simulink model "generic_IVS"  (R2024a)
settings: Solver=FixedStepDiscrete  StartTime=0.0  StopTime=inf  FixedStep=0.001  RelTol=1e-3  EnableMultiTasking=on
libraries: CarMaker4SL x57, simulink x1, slpidlib x1
(part 3 of 4)

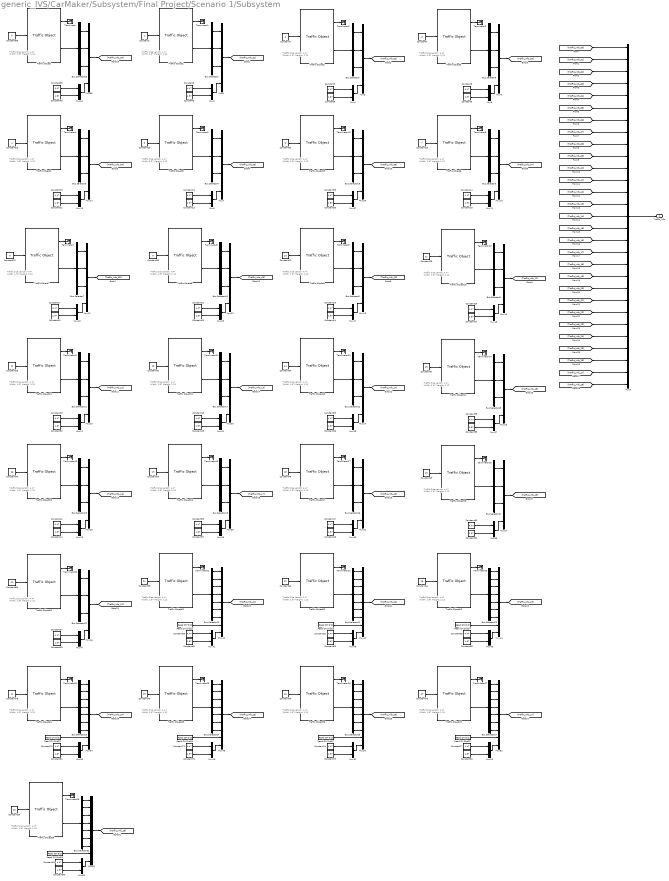
== system generic_IVS/CarMaker/Subsystem/Final Project/Scenario 1/Subsystem ==
  note: Traffic Size
      | Length: 4.47
      | Width: 1.97
      | Height: 1.12
  note: Traffic Size
      | Length: 4.47
      | Width: 1.97
      | Height: 1.12
  note: Traffic Size
      | Length: 4.47
      | Width: 1.97
      | Height: 1.12
  note: Traffic Size
      | Length: 4.47
      | Width: 1.97
      | Height: 1.12
  note: Traffic Size
      | Length: 4.47
      | Width: 1.97
      | Height: 1.12
  note: Traffic Size
      | Length: 4.47
      | Width: 1.97
      | Height: 1.12
  note: Traffic Size
      | Length: 4.47
      | Width: 1.97
      | Height: 1.12
  note: Traffic Size
      | Length: 4.47
      | Width: 1.97
      | Height: 1.12
  note: Traffic Size
      | Length: 4.47
      | Width: 1.97
      | Height: 1.12
  note: Traffic Size
      | Length: 4.47
      | Width: 1.97
      | Height: 1.12
  note: Traffic Size
      | Length: 4.47
      | Width: 1.97
      | Height: 1.12
  note: Traffic Size
      | Length: 4.47
      | Width: 1.97
      | Height: 1.12
  note: Traffic Size
      | Length: 4.47
      | Width: 1.97
      | Height: 1.12
  note: Traffic Size
      | Length: 4.47
      | Width: 1.97
      | Height: 1.12
  note: Traffic Size
      | Length: 4.47
      | Width: 1.97
      | Height: 1.12
  note: Traffic Size
      | Length: 4.47
      | Width: 1.97
      | Height: 1.12
  note: Traffic Size
      | Length: 4.47
      | Width: 1.97
      | Height: 1.12
  note: Traffic Size
      | Length: 4.47
      | Width: 1.97
      | Height: 1.12
  note: Traffic Size
      | Length: 4.47
      | Width: 1.97
      | Height: 1.12
  note: Traffic Size
      | Length: 4.47
      | Width: 1.97
      | Height: 1.12
  note: Traffic Size
      | Length: 4.47
      | Width: 1.97
      | Height: 1.12
  note: Traffic Size
      | Length: 4.47
      | Width: 1.97
      | Height: 1.12
  note: Traffic Size
      | Length: 4.47
      | Width: 1.97
      | Height: 1.12
  note: Traffic Size
      | Length: 4.47
      | Width: 1.97
      | Height: 1.12
  note: Traffic Size
      | Length: 4.47
      | Width: 1.97
      | Height: 1.12
  note: Traffic Size
      | Length: 4.47
      | Width: 1.97
      | Height: 1.12
  note: Traffic Size
      | Length: 4.47
      | Width: 1.97
      | Height: 1.12
  note: Traffic Size
      | Length: 4.47
      | Width: 1.97
      | Height: 1.12
  note: Traffic Size
      | Length: 4.47
      | Width: 1.97
      | Height: 1.12
  Bus Selector{1..19,22,29} (21 alike) : BusSelector  OutputSignals=t_0 x,t_0 y,r_zyx z
  Bus Selector{20..21,23..27,31} (8 alike) : BusSelector  OutputSignals=t_0 x,t_0 y,v_0 x,v_0 y,a_0 x,a_0 y,r_zyx z
  Constant1 : Constant
  Constant10 : Constant  Value=5
  Constant{2,5,8,11,14,17,19,23,26,29,31,35,38,41,43,47,50,53,55,59,62,65,67,71,74,77,79,89,94} (29 alike) : Constant  Value=4.47
  Constant{3,6,9,12,15,20..21,24,27,32..33,36,39,44..45,48,51,56..57,60,63,68..69,72,75,80..81,90,96} (29 alike) : Constant  Value=1.97
  Constant13 : Constant  Value=7
  Constant16 : Constant  Value=8
  Constant18 : Constant  Value=4
  Constant22 : Constant  Value=10
  Constant25 : Constant  Value=11
  Constant28 : Constant  Value=12
  Constant30 : Constant  Value=9
  Constant34 : Constant  Value=14
  Constant37 : Constant  Value=15
  Constant4 : Constant  Value=2
  Constant40 : Constant  Value=16
  Constant42 : Constant  Value=13
  Constant46 : Constant  Value=18
  Constant49 : Constant  Value=19
  Constant52 : Constant  Value=6
  Constant54 : Constant  Value=17
  Constant58 : Constant  Value=21
  Constant61 : Constant  Value=22
  Constant64 : Constant  Value=23
  Constant66 : Constant  Value=20
  Constant7 : Constant  Value=3
  Constant70 : Constant  Value=25
  Constant73 : Constant  Value=26
  Constant76 : Constant  Value=27
  Constant78 : Constant  Value=24
  Constant88 : Constant  Value=0
  Constant93 : Constant  Value=28
  Mux{1,3,5,7,10,12,14,16,18,20,22,24,26,28,30,32,34,36,38,46,60} (21 alike) : Mux
  Mux{2,4,6,8,11,13,15,17,19,21,23,25,27,29,31,33,35,37,39,41,43,45,47,49,51,53,55,61,65} (29 alike) : Mux  Inputs=2
  Mux{40,42,44,48,50,52,54,64} (8 alike) : Mux  Inputs=9
  Mux9 : Mux  Inputs=29
  Read CM Dict22 : CarMaker4SL/Read CM Dict  xname=Traffic.T21.rzv  xsync=off  xstime=Inherited
  Read CM Dict23 : CarMaker4SL/Read CM Dict  xname=Traffic.T22.rzv  xsync=off  xstime=Inherited
  Read CM Dict24 : CarMaker4SL/Read CM Dict  xname=Traffic.T23.rzv  xsync=off  xstime=Inherited
  Read CM Dict25 : CarMaker4SL/Read CM Dict  xname=Traffic.T24.rzv  xsync=off  xstime=Inherited
  Read CM Dict26 : CarMaker4SL/Read CM Dict  xname=Traffic.T25.rzv  xsync=off  xstime=Inherited
  Read CM Dict27 : CarMaker4SL/Read CM Dict  xname=Traffic.T26.rzv  xsync=off  xstime=Inherited
  Read CM Dict28 : CarMaker4SL/Read CM Dict  xname=Traffic.T27.rzv  xsync=off  xstime=Inherited
  Read CM Dict29 : CarMaker4SL/Read CM Dict  xname=Traffic.T28.rzv  xsync=off  xstime=Inherited
  Terminator{,1..28} (29 alike) : Terminator
  Traffic Object : CarMaker4SL/Traffic Object  xname=T00  ximode=Traffic Id  xstime=Inherited
      settings: SourceProductName=CarMaker4SL
  Traffic Object1 : CarMaker4SL/Traffic Object  xname=T01  ximode=Traffic Id  xstime=Inherited
      settings: SourceProductName=CarMaker4SL
  Traffic Object10 : CarMaker4SL/Traffic Object  xname=T11  ximode=Traffic Id  xstime=Inherited
      settings: SourceProductName=CarMaker4SL
  Traffic Object11 : CarMaker4SL/Traffic Object  xname=T12  ximode=Traffic Id  xstime=Inherited
      settings: SourceProductName=CarMaker4SL
  Traffic Object12 : CarMaker4SL/Traffic Object  xname=T13  ximode=Traffic Id  xstime=Inherited
      settings: SourceProductName=CarMaker4SL
  Traffic Object13 : CarMaker4SL/Traffic Object  xname=T14  ximode=Traffic Id  xstime=Inherited
      settings: SourceProductName=CarMaker4SL
  Traffic Object14 : CarMaker4SL/Traffic Object  xname=T15  ximode=Traffic Id  xstime=Inherited
      settings: SourceProductName=CarMaker4SL
  Traffic Object15 : CarMaker4SL/Traffic Object  xname=T16  ximode=Traffic Id  xstime=Inherited
      settings: SourceProductName=CarMaker4SL
  Traffic Object16 : CarMaker4SL/Traffic Object  xname=T17  ximode=Traffic Id  xstime=Inherited
      settings: SourceProductName=CarMaker4SL
  Traffic Object17 : CarMaker4SL/Traffic Object  xname=T18  ximode=Traffic Id  xstime=Inherited
      settings: SourceProductName=CarMaker4SL
  Traffic Object18 : CarMaker4SL/Traffic Object  xname=T19  ximode=Traffic Id  xstime=Inherited
      settings: SourceProductName=CarMaker4SL
  Traffic Object19 : CarMaker4SL/Traffic Object  xname=T06  ximode=Traffic Id  xstime=Inherited
      settings: SourceProductName=CarMaker4SL
  Traffic Object2 : CarMaker4SL/Traffic Object  xname=T02  ximode=Traffic Id  xstime=Inherited
      settings: SourceProductName=CarMaker4SL
  Traffic Object20 : CarMaker4SL/Traffic Object  xname=T20  ximode=Traffic Id  xstime=Inherited
      settings: SourceProductName=CarMaker4SL
  Traffic Object21 : CarMaker4SL/Traffic Object  xname=T21  ximode=Traffic Id  xstime=Inherited
      settings: SourceProductName=CarMaker4SL
  Traffic Object22 : CarMaker4SL/Traffic Object  xname=T22  ximode=Traffic Id  xstime=Inherited
      settings: SourceProductName=CarMaker4SL
  Traffic Object23 : CarMaker4SL/Traffic Object  xname=T23  ximode=Traffic Id  xstime=Inherited
      settings: SourceProductName=CarMaker4SL
  Traffic Object24 : CarMaker4SL/Traffic Object  xname=T24  ximode=Traffic Id  xstime=Inherited
      settings: SourceProductName=CarMaker4SL
  Traffic Object25 : CarMaker4SL/Traffic Object  xname=T25  ximode=Traffic Id  xstime=Inherited
      settings: SourceProductName=CarMaker4SL
  Traffic Object26 : CarMaker4SL/Traffic Object  xname=T26  ximode=Traffic Id  xstime=Inherited
      settings: SourceProductName=CarMaker4SL
  Traffic Object27 : CarMaker4SL/Traffic Object  xname=T27  ximode=Traffic Id  xstime=Inherited
      settings: SourceProductName=CarMaker4SL
  Traffic Object28 : CarMaker4SL/Traffic Object  xname=T28  ximode=Traffic Id  xstime=Inherited
      settings: SourceProductName=CarMaker4SL
  Traffic Object3 : CarMaker4SL/Traffic Object  xname=T03  ximode=Traffic Id  xstime=Inherited
      settings: SourceProductName=CarMaker4SL
  Traffic Object4 : CarMaker4SL/Traffic Object  xname=T04  ximode=Traffic Id  xstime=Inherited
      settings: SourceProductName=CarMaker4SL
  Traffic Object5 : CarMaker4SL/Traffic Object  xname=T05  ximode=Traffic Id  xstime=Inherited
      settings: SourceProductName=CarMaker4SL
  Traffic Object6 : CarMaker4SL/Traffic Object  xname=T07  ximode=Traffic Id  xstime=Inherited
      settings: SourceProductName=CarMaker4SL
  Traffic Object7 : CarMaker4SL/Traffic Object  xname=T08  ximode=Traffic Id  xstime=Inherited
      settings: SourceProductName=CarMaker4SL
  Traffic Object8 : CarMaker4SL/Traffic Object  xname=T09  ximode=Traffic Id  xstime=Inherited
      settings: SourceProductName=CarMaker4SL
  Traffic Object9 : CarMaker4SL/Traffic Object  xname=T10  ximode=Traffic Id  xstime=Inherited
      settings: SourceProductName=CarMaker4SL
  Traffic_Info : Outport
  wires:
  [Traffic_Info_00] -> Mux9/1
  [Traffic_Info_01] -> Mux9/2
  Mux9/1 -> Traffic_Info/1
  [Traffic_Info_02] -> Mux9/3
  [Traffic_Info_06] -> Mux9/7
  [Traffic_Info_05] -> Mux9/6
  [Traffic_Info_04] -> Mux9/5
  [Traffic_Info_03] -> Mux9/4
  [Traffic_Info_09] -> Mux9/10
  [Traffic_Info_10] -> Mux9/11
  [Traffic_Info_11] -> Mux9/12
  [Traffic_Info_08] -> Mux9/9
  [Traffic_Info_12] -> Mux9/13
  [Traffic_Info_13] -> Mux9/14
  [Traffic_Info_07] -> Mux9/8
  [Traffic_Info_16] -> Mux9/17
  [Traffic_Info_17] -> Mux9/18
  [Traffic_Info_18] -> Mux9/19
  [Traffic_Info_15] -> Mux9/16
  [Traffic_Info_19] -> Mux9/20
  [Traffic_Info_20] -> Mux9/21
  [Traffic_Info_14] -> Mux9/15
  [Traffic_Info_23] -> Mux9/24
  [Traffic_Info_24] -> Mux9/25
  [Traffic_Info_25] -> Mux9/26
  [Traffic_Info_22] -> Mux9/23
  [Traffic_Info_26] -> Mux9/27
  [Traffic_Info_27] -> Mux9/28
  [Traffic_Info_21] -> Mux9/22
  [Traffic_Info_28] -> Mux9/29
  Traffic Object/2 -> Bus Selector29/1
  Constant88/1 -> Traffic Object/1
  Traffic Object/1 -> Terminator/1
  Bus Selector29/1 -> Mux60/1  "<t_0 x>"
  Bus Selector29/2 -> Mux60/2  "<t_0 y>"
  Bus Selector29/3 -> Mux60/3  "<r_zyx z>"
  Mux60/1 -> [Traffic_Info_00]
  Constant89/1 -> Mux61/1
  Constant90/1 -> Mux61/2
  Mux61/1 -> Mux60/4
  Bus Selector23/5 -> Mux44/5  "<a_0 x>"
  Traffic Object22/2 -> Bus Selector21/1
  Mux41/1 -> Mux40/9
  Constant63/1 -> Mux43/2
  Bus Selector23/2 -> Mux44/2  "<t_0 y>"
  Bus Selector21/2 -> Mux42/2  "<t_0 y>"
  Bus Selector21/5 -> Mux42/5  "<a_0 x>"
  Traffic Object22/1 -> Terminator22/1
  Bus Selector23/6 -> Mux44/6  "<a_0 y>"
  Bus Selector23/7 -> Mux44/7  "<r_zyx z>"
  Traffic Object23/1 -> Terminator23/1
  Traffic Object23/2 -> Bus Selector23/1
  Constant68/1 -> Mux45/2
  Mux45/1 -> Mux44/9
  Constant61/1 -> Traffic Object22/1
  Read CM Dict24/1 -> Mux44/8
  Mux42/1 -> [Traffic_Info_22]
  Mux40/1 -> [Traffic_Info_21]
  Mux44/1 -> [Traffic_Info_23]
  Bus Selector23/4 -> Mux44/4  "<v_0 y>"
  Bus Selector21/6 -> Mux42/6  "<a_0 y>"
  Bus Selector20/6 -> Mux40/6  "<a_0 y>"
  Bus Selector21/3 -> Mux42/3  "<v_0 x>"
  Bus Selector21/4 -> Mux42/4  "<v_0 y>"
  Bus Selector21/1 -> Mux42/1  "<t_0 x>"
  Constant58/1 -> Traffic Object21/1
  Bus Selector21/7 -> Mux42/7  "<r_zyx z>"
  Constant65/1 -> Mux45/1
  Bus Selector20/1 -> Mux40/1  "<t_0 x>"
  Bus Selector23/1 -> Mux44/1  "<t_0 x>"
  Bus Selector20/3 -> Mux40/3  "<v_0 x>"
  Constant60/1 -> Mux41/2
  Traffic Object21/2 -> Bus Selector20/1
  Read CM Dict22/1 -> Mux40/8
  Bus Selector20/5 -> Mux40/5  "<a_0 x>"
  Traffic Object21/1 -> Terminator21/1
  Bus Selector20/2 -> Mux40/2  "<t_0 y>"
  Bus Selector23/3 -> Mux44/3  "<v_0 x>"
  Constant64/1 -> Traffic Object23/1
  Bus Selector20/7 -> Mux40/7  "<r_zyx z>"
  Read CM Dict23/1 -> Mux42/8
  Constant62/1 -> Mux43/1
  Bus Selector20/4 -> Mux40/4  "<v_0 y>"
  Constant59/1 -> Mux41/1
  Mux43/1 -> Mux42/9
  Bus Selector26/3 -> Mux54/3  "<v_0 x>"
  Bus Selector27/5 -> Mux52/5  "<a_0 x>"
  Bus Selector26/5 -> Mux54/5  "<a_0 x>"
  Traffic Object26/2 -> Bus Selector25/1
  Bus Selector26/6 -> Mux54/6  "<a_0 y>"
  Mux49/1 -> Mux48/9
  Constant75/1 -> Mux51/2
  Bus Selector27/2 -> Mux52/2  "<t_0 y>"
  Bus Selector25/2 -> Mux50/2  "<t_0 y>"
  Bus Selector25/5 -> Mux50/5  "<a_0 x>"
  Traffic Object26/1 -> Terminator26/1
  Bus Selector27/6 -> Mux52/6  "<a_0 y>"
  Bus Selector26/7 -> Mux54/7  "<r_zyx z>"
  Bus Selector27/7 -> Mux52/7  "<r_zyx z>"
  Bus Selector26/1 -> Mux54/1  "<t_0 x>"
  Traffic Object27/1 -> Terminator27/1
  Traffic Object27/2 -> Bus Selector27/1
  Constant80/1 -> Mux53/2
  Mux53/1 -> Mux52/9
  Constant73/1 -> Traffic Object26/1
  Read CM Dict28/1 -> Mux52/8
  Mux50/1 -> [Traffic_Info_26]
  Mux48/1 -> [Traffic_Info_25]
  Mux52/1 -> [Traffic_Info_27]
  Bus Selector27/4 -> Mux52/4  "<v_0 y>"
  Constant78/1 -> Traffic Object24/1
  Traffic Object24/1 -> Terminator24/1
  Bus Selector25/6 -> Mux50/6  "<a_0 y>"
  Bus Selector24/6 -> Mux48/6  "<a_0 y>"
  Bus Selector25/3 -> Mux50/3  "<v_0 x>"
  Read CM Dict25/1 -> Mux54/8
  Bus Selector25/4 -> Mux50/4  "<v_0 y>"
  Bus Selector26/4 -> Mux54/4  "<v_0 y>"
  Bus Selector25/1 -> Mux50/1  "<t_0 x>"
  Constant70/1 -> Traffic Object25/1
  Bus Selector25/7 -> Mux50/7  "<r_zyx z>"
  Constant77/1 -> Mux53/1
  Bus Selector26/2 -> Mux54/2  "<t_0 y>"
  Bus Selector24/1 -> Mux48/1  "<t_0 x>"
  Bus Selector27/1 -> Mux52/1  "<t_0 x>"
  Bus Selector24/3 -> Mux48/3  "<v_0 x>"
  Mux54/1 -> [Traffic_Info_24]
  Constant72/1 -> Mux49/2
  Traffic Object25/2 -> Bus Selector24/1
  Read CM Dict26/1 -> Mux48/8
  Bus Selector24/5 -> Mux48/5  "<a_0 x>"
  Traffic Object25/1 -> Terminator25/1
  Constant81/1 -> Mux55/2
  Bus Selector24/2 -> Mux48/2  "<t_0 y>"
  Bus Selector27/3 -> Mux52/3  "<v_0 x>"
  Constant76/1 -> Traffic Object27/1
  Bus Selector24/7 -> Mux48/7  "<r_zyx z>"
  Traffic Object24/2 -> Bus Selector26/1
  Read CM Dict27/1 -> Mux50/8
  Mux55/1 -> Mux54/9
  Constant74/1 -> Mux51/1
  Bus Selector24/4 -> Mux48/4  "<v_0 y>"
  Constant71/1 -> Mux49/1
  Constant79/1 -> Mux55/1
  Mux51/1 -> Mux50/9
  Bus Selector31/3 -> Mux64/3  "<v_0 x>"
  Bus Selector31/5 -> Mux64/5  "<a_0 x>"
  Bus Selector31/6 -> Mux64/6  "<a_0 y>"
  Bus Selector31/7 -> Mux64/7  "<r_zyx z>"
  Bus Selector31/1 -> Mux64/1  "<t_0 x>"
  Constant93/1 -> Traffic Object28/1
  Traffic Object28/1 -> Terminator28/1
  Read CM Dict29/1 -> Mux64/8
  Bus Selector31/4 -> Mux64/4  "<v_0 y>"
  Bus Selector31/2 -> Mux64/2  "<t_0 y>"
  Mux64/1 -> [Traffic_Info_28]
  Constant96/1 -> Mux65/2
  Traffic Object28/2 -> Bus Selector31/1
  Mux65/1 -> Mux64/9
  Constant94/1 -> Mux65/1
  Bus Selector1/3 -> Mux1/3  "<r_zyx z>"
  Mux1/1 -> [Traffic_Info_01]
  Bus Selector1/1 -> Mux1/1  "<t_0 x>"
  Traffic Object1/1 -> Terminator1/1
  Constant2/1 -> Mux2/1
  Constant3/1 -> Mux2/2
  Bus Selector1/2 -> Mux1/2  "<t_0 y>"
  Mux2/1 -> Mux1/4
  Constant1/1 -> Traffic Object1/1
  Traffic Object1/2 -> Bus Selector1/1
  Bus Selector2/3 -> Mux3/3  "<r_zyx z>"
  Mux3/1 -> [Traffic_Info_02]
  Bus Selector2/1 -> Mux3/1  "<t_0 x>"
  Traffic Object2/1 -> Terminator2/1
  Constant5/1 -> Mux4/1
  Constant6/1 -> Mux4/2
  Bus Selector2/2 -> Mux3/2  "<t_0 y>"
  Mux4/1 -> Mux3/4
  Constant4/1 -> Traffic Object2/1
  Traffic Object2/2 -> Bus Selector2/1
  Bus Selector3/3 -> Mux5/3  "<r_zyx z>"
  Mux5/1 -> [Traffic_Info_03]
  Bus Selector3/1 -> Mux5/1  "<t_0 x>"
  Traffic Object3/1 -> Terminator3/1
  Constant8/1 -> Mux6/1
  Constant9/1 -> Mux6/2
  Bus Selector3/2 -> Mux5/2  "<t_0 y>"
  Mux6/1 -> Mux5/4
  Constant7/1 -> Traffic Object3/1
  Traffic Object3/2 -> Bus Selector3/1
  Bus Selector6/3 -> Mux14/3  "<r_zyx z>"
  Mux14/1 -> [Traffic_Info_04]
  Bus Selector6/1 -> Mux14/1  "<t_0 x>"
  Mux8/1 -> Mux7/4
  Constant12/1 -> Mux8/2
  Mux7/1 -> [Traffic_Info_05]
  Traffic Object4/1 -> Terminator4/1
  Bus Selector4/2 -> Mux7/2  "<t_0 y>"
  Constant18/1 -> Traffic Object4/1
  Constant21/1 -> Mux15/2
  Constant10/1 -> Traffic Object5/1
  Bus Selector6/2 -> Mux14/2  "<t_0 y>"
  Mux15/1 -> Mux14/4
  Traffic Object4/2 -> Bus Selector6/1
  Constant16/1 -> Traffic Object7/1
  Traffic Object7/2 -> Bus Selector7/1
  Constant17/1 -> Mux13/1
  Constant19/1 -> Mux15/1
  Constant11/1 -> Mux8/1
  Traffic Object7/1 -> Terminator7/1
  Constant20/1 -> Mux13/2
  Bus Selector4/1 -> Mux7/1  "<t_0 x>"
  Mux13/1 -> Mux12/4
  Bus Selector7/1 -> Mux12/1  "<t_0 x>"
  Bus Selector4/3 -> Mux7/3  "<r_zyx z>"
  Bus Selector7/3 -> Mux12/3  "<r_zyx z>"
  Mux12/1 -> [Traffic_Info_08]
  Constant15/1 -> Mux11/2
  Mux11/1 -> Mux10/4
  Constant13/1 -> Traffic Object6/1
  Traffic Object5/1 -> Terminator5/1
  Constant14/1 -> Mux11/1
  Traffic Object6/1 -> Terminator6/1
  Traffic Object5/2 -> Bus Selector4/1
  Bus Selector5/1 -> Mux10/1  "<t_0 x>"
  Bus Selector7/2 -> Mux12/2  "<t_0 y>"
  Traffic Object6/2 -> Bus Selector5/1
  Bus Selector5/3 -> Mux10/3  "<r_zyx z>"
  Mux10/1 -> [Traffic_Info_07]
  Bus Selector5/2 -> Mux10/2  "<t_0 y>"
  Bus Selector10/3 -> Mux22/3  "<r_zyx z>"
  Mux22/1 -> [Traffic_Info_09]
  Bus Selector10/1 -> Mux22/1  "<t_0 x>"
  Mux17/1 -> Mux16/4
  Constant24/1 -> Mux17/2
  Mux16/1 -> [Traffic_Info_10]
  Traffic Object8/1 -> Terminator8/1
  Bus Selector8/2 -> Mux16/2  "<t_0 y>"
  Constant30/1 -> Traffic Object8/1
  Constant33/1 -> Mux23/2
  Constant22/1 -> Traffic Object9/1
  Bus Selector10/2 -> Mux22/2  "<t_0 y>"
  Mux23/1 -> Mux22/4
  Traffic Object8/2 -> Bus Selector10/1
  Constant28/1 -> Traffic Object11/1
  Traffic Object11/2 -> Bus Selector11/1
  Constant29/1 -> Mux21/1
  Constant31/1 -> Mux23/1
  Constant23/1 -> Mux17/1
  Traffic Object11/1 -> Terminator11/1
  Constant32/1 -> Mux21/2
  Bus Selector8/1 -> Mux16/1  "<t_0 x>"
  Mux21/1 -> Mux20/4
  Bus Selector11/1 -> Mux20/1  "<t_0 x>"
  Bus Selector8/3 -> Mux16/3  "<r_zyx z>"
  Bus Selector11/3 -> Mux20/3  "<r_zyx z>"
  Mux20/1 -> [Traffic_Info_12]
  Constant27/1 -> Mux19/2
  Mux19/1 -> Mux18/4
  Constant25/1 -> Traffic Object10/1
  Traffic Object9/1 -> Terminator9/1
  Constant26/1 -> Mux19/1
  Traffic Object10/1 -> Terminator10/1
  Traffic Object9/2 -> Bus Selector8/1
  Bus Selector9/1 -> Mux18/1  "<t_0 x>"
  Bus Selector11/2 -> Mux20/2  "<t_0 y>"
  Traffic Object10/2 -> Bus Selector9/1
  Bus Selector9/3 -> Mux18/3  "<r_zyx z>"
  Mux18/1 -> [Traffic_Info_11]
  Bus Selector9/2 -> Mux18/2  "<t_0 y>"
  Bus Selector14/3 -> Mux30/3  "<r_zyx z>"
  Mux30/1 -> [Traffic_Info_13]
  Bus Selector14/1 -> Mux30/1  "<t_0 x>"
  Mux25/1 -> Mux24/4
  Constant36/1 -> Mux25/2
  Mux24/1 -> [Traffic_Info_14]
  Traffic Object12/1 -> Terminator12/1
  Bus Selector12/2 -> Mux24/2  "<t_0 y>"
  Constant42/1 -> Traffic Object12/1
  Constant45/1 -> Mux31/2
  Constant34/1 -> Traffic Object13/1
  Bus Selector14/2 -> Mux30/2  "<t_0 y>"
  Mux31/1 -> Mux30/4
  Traffic Object12/2 -> Bus Selector14/1
  Constant40/1 -> Traffic Object15/1
  Traffic Object15/2 -> Bus Selector15/1
  Constant41/1 -> Mux29/1
  Constant43/1 -> Mux31/1
  Constant35/1 -> Mux25/1
  Traffic Object15/1 -> Terminator15/1
  Constant44/1 -> Mux29/2
  Bus Selector12/1 -> Mux24/1  "<t_0 x>"
  Mux29/1 -> Mux28/4
  Bus Selector15/1 -> Mux28/1  "<t_0 x>"
  Bus Selector12/3 -> Mux24/3  "<r_zyx z>"
  Bus Selector15/3 -> Mux28/3  "<r_zyx z>"
  Mux28/1 -> [Traffic_Info_16]
  Constant39/1 -> Mux27/2
  Mux27/1 -> Mux26/4
  Constant37/1 -> Traffic Object14/1
  Traffic Object13/1 -> Terminator13/1
  Constant38/1 -> Mux27/1
  Traffic Object14/1 -> Terminator14/1
  Traffic Object13/2 -> Bus Selector12/1
  Bus Selector13/1 -> Mux26/1  "<t_0 x>"
  Bus Selector15/2 -> Mux28/2  "<t_0 y>"
  Traffic Object14/2 -> Bus Selector13/1
  Bus Selector13/3 -> Mux26/3  "<r_zyx z>"
  Mux26/1 -> [Traffic_Info_15]
  Bus Selector13/2 -> Mux26/2  "<t_0 y>"
  Bus Selector17/1 -> Mux34/1  "<t_0 x>"
  Traffic Object18/1 -> Terminator18/1
  Constant49/1 -> Traffic Object18/1
  Traffic Object17/2 -> Bus Selector16/1
  Traffic Object17/1 -> Terminator17/1
  Mux34/1 -> [Traffic_Info_19]
  Bus Selector17/3 -> Mux34/3  "<r_zyx z>"
  Constant50/1 -> Mux35/1
  Constant51/1 -> Mux35/2
  Traffic Object18/2 -> Bus Selector17/1
  Constant55/1 -> Mux39/1
  Bus Selector17/2 -> Mux34/2  "<t_0 y>"
  Constant47/1 -> Mux33/1
  Bus Selector16/1 -> Mux32/1  "<t_0 x>"
  Bus Selector16/3 -> Mux32/3  "<r_zyx z>"
  Traffic Object16/2 -> Bus Selector18/1
  Mux39/1 -> Mux38/4
  Constant46/1 -> Traffic Object17/1
  Mux35/1 -> Mux34/4
  Mux32/1 -> [Traffic_Info_18]
  Constant54/1 -> Traffic Object16/1
  Traffic Object16/1 -> Terminator16/1
  Constant48/1 -> Mux33/2
  Mux33/1 -> Mux32/4
  Constant57/1 -> Mux39/2
  Bus Selector18/1 -> Mux38/1  "<t_0 x>"
  Bus Selector18/3 -> Mux38/3  "<r_zyx z>"
  Bus Selector16/2 -> Mux32/2  "<t_0 y>"
  Mux38/1 -> [Traffic_Info_17]
  Bus Selector18/2 -> Mux38/2  "<t_0 y>"
  Bus Selector19/1 -> Mux36/1  "<t_0 x>"
  Traffic Object19/1 -> Terminator19/1
  Constant53/1 -> Mux37/1
  Bus Selector19/2 -> Mux36/2  "<t_0 y>"
  Mux36/1 -> [Traffic_Info_06]
  Bus Selector19/3 -> Mux36/3  "<r_zyx z>"
  Traffic Object19/2 -> Bus Selector19/1
  Mux37/1 -> Mux36/4
  Constant52/1 -> Traffic Object19/1
  Constant56/1 -> Mux37/2
  Constant69/1 -> Mux47/2
  Traffic Object20/2 -> Bus Selector22/1
  Bus Selector22/2 -> Mux46/2  "<t_0 y>"
  Bus Selector22/3 -> Mux46/3  "<r_zyx z>"
  Mux46/1 -> [Traffic_Info_20]
  Constant67/1 -> Mux47/1
  Mux47/1 -> Mux46/4
  Bus Selector22/1 -> Mux46/1  "<t_0 x>"
  Constant66/1 -> Traffic Object20/1
  Traffic Object20/1 -> Terminator20/1

== system generic_IVS/CarMaker/IPG Vehicle/CarAndTrailer/Forces/Suspension Forces/Suspension External Forces Update ==
  Bus Creator21 : BusCreator  Inputs=6
  Bus Creator22 : BusCreator  Inputs=4
  Bus Creator23 : BusCreator  Inputs=4
  From : From  TagVisibility=global
  Ground{32..39} (8 alike) : Ground
  Out1 : Outport
  wires:
  [D] -> Bus Creator21/4
  Ground36/1 -> Bus Creator22/1
  From/1 -> Bus Creator21/1
  [B] -> Bus Creator21/2
  Ground34/1 -> Bus Creator23/3
  Ground32/1 -> Bus Creator23/1
  [C] -> Bus Creator21/3
  Bus Creator23/1 -> Bus Creator21/5
  Ground33/1 -> Bus Creator23/2
  Bus Creator22/1 -> Bus Creator21/6
  Bus Creator21/1 -> Out1/1
  Ground35/1 -> Bus Creator23/4
  Ground39/1 -> Bus Creator22/4
  Ground38/1 -> Bus Creator22/3
  Ground37/1 -> Bus Creator22/2

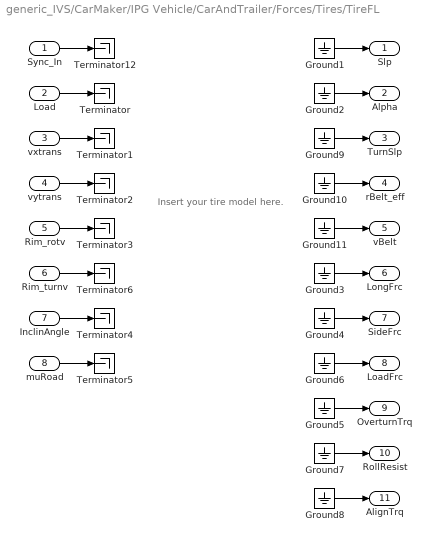
== system generic_IVS/CarMaker/IPG Vehicle/CarAndTrailer/Forces/Tires/TireFL ==
  note: Insert your tire model here.
  Sync_In : Inport
  Load : Inport  Port=2
  vxtrans : Inport  Port=3
  vytrans : Inport  Port=4
  Rim_rotv : Inport  Port=5
  Rim_turnv : Inport  Port=6
  InclinAngle : Inport  Port=7
  muRoad : Inport  Port=8
  Ground{1..11} (11 alike) : Ground
  Terminator{,1..6,12} (8 alike) : Terminator
  Slp : Outport  VectorParamsAs1DForOutWhenUnconnected=off
  Alpha : Outport  Port=2  VectorParamsAs1DForOutWhenUnconnected=off
  TurnSlp : Outport  Port=3  VectorParamsAs1DForOutWhenUnconnected=off
  rBelt_eff : Outport  Port=4  VectorParamsAs1DForOutWhenUnconnected=off
  vBelt : Outport  Port=5  VectorParamsAs1DForOutWhenUnconnected=off
  LongFrc : Outport  Port=6  VectorParamsAs1DForOutWhenUnconnected=off
  SideFrc : Outport  Port=7  VectorParamsAs1DForOutWhenUnconnected=off
  LoadFrc : Outport  Port=8  VectorParamsAs1DForOutWhenUnconnected=off
  OverturnTrq : Outport  Port=9  VectorParamsAs1DForOutWhenUnconnected=off
  RollResist : Outport  Port=10  VectorParamsAs1DForOutWhenUnconnected=off
  AlignTrq : Outport  Port=11  VectorParamsAs1DForOutWhenUnconnected=off
  wires:
  Ground11/1 -> vBelt/1
  Ground10/1 -> rBelt_eff/1
  Ground9/1 -> TurnSlp/1
  Rim_turnv/1 -> Terminator6/1
  Sync_In/1 -> Terminator12/1
  Ground2/1 -> Alpha/1
  Ground3/1 -> LongFrc/1
  Ground4/1 -> SideFrc/1
  Ground5/1 -> OverturnTrq/1
  vxtrans/1 -> Terminator1/1
  vytrans/1 -> Terminator2/1
  Rim_rotv/1 -> Terminator3/1
  InclinAngle/1 -> Terminator4/1
  muRoad/1 -> Terminator5/1
  Load/1 -> Terminator/1
  Ground1/1 -> Slp/1
  Ground6/1 -> LoadFrc/1
  Ground7/1 -> RollResist/1
  Ground8/1 -> AlignTrq/1

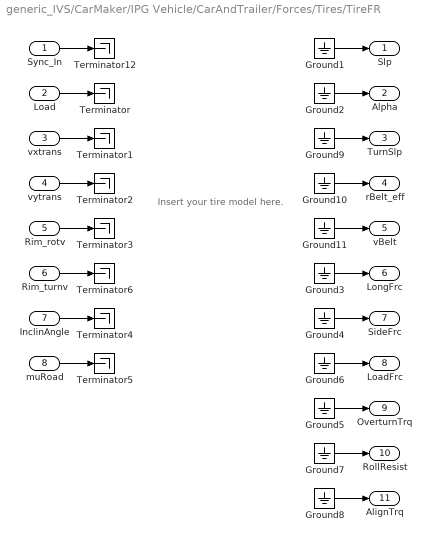
== system generic_IVS/CarMaker/IPG Vehicle/CarAndTrailer/Forces/Tires/TireFR ==
  note: Insert your tire model here.
  Sync_In : Inport
  Load : Inport  Port=2
  vxtrans : Inport  Port=3
  vytrans : Inport  Port=4
  Rim_rotv : Inport  Port=5
  Rim_turnv : Inport  Port=6
  InclinAngle : Inport  Port=7
  muRoad : Inport  Port=8
  Ground{1..11} (11 alike) : Ground
  Terminator{,1..6,12} (8 alike) : Terminator
  Slp : Outport  VectorParamsAs1DForOutWhenUnconnected=off
  Alpha : Outport  Port=2  VectorParamsAs1DForOutWhenUnconnected=off
  TurnSlp : Outport  Port=3  VectorParamsAs1DForOutWhenUnconnected=off
  rBelt_eff : Outport  Port=4  VectorParamsAs1DForOutWhenUnconnected=off
  vBelt : Outport  Port=5  VectorParamsAs1DForOutWhenUnconnected=off
  LongFrc : Outport  Port=6  VectorParamsAs1DForOutWhenUnconnected=off
  SideFrc : Outport  Port=7  VectorParamsAs1DForOutWhenUnconnected=off
  LoadFrc : Outport  Port=8  VectorParamsAs1DForOutWhenUnconnected=off
  OverturnTrq : Outport  Port=9  VectorParamsAs1DForOutWhenUnconnected=off
  RollResist : Outport  Port=10  VectorParamsAs1DForOutWhenUnconnected=off
  AlignTrq : Outport  Port=11  VectorParamsAs1DForOutWhenUnconnected=off
  wires:
  Ground11/1 -> vBelt/1
  Ground10/1 -> rBelt_eff/1
  Ground9/1 -> TurnSlp/1
  Rim_turnv/1 -> Terminator6/1
  Sync_In/1 -> Terminator12/1
  Ground2/1 -> Alpha/1
  Ground3/1 -> LongFrc/1
  Ground4/1 -> SideFrc/1
  Ground5/1 -> OverturnTrq/1
  vxtrans/1 -> Terminator1/1
  vytrans/1 -> Terminator2/1
  Rim_rotv/1 -> Terminator3/1
  InclinAngle/1 -> Terminator4/1
  muRoad/1 -> Terminator5/1
  Load/1 -> Terminator/1
  Ground1/1 -> Slp/1
  Ground6/1 -> LoadFrc/1
  Ground7/1 -> RollResist/1
  Ground8/1 -> AlignTrq/1

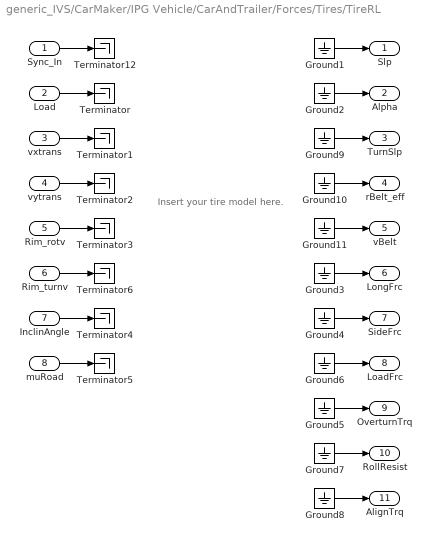
== system generic_IVS/CarMaker/IPG Vehicle/CarAndTrailer/Forces/Tires/TireRL ==
  note: Insert your tire model here.
  Sync_In : Inport
  Load : Inport  Port=2
  vxtrans : Inport  Port=3
  vytrans : Inport  Port=4
  Rim_rotv : Inport  Port=5
  Rim_turnv : Inport  Port=6
  InclinAngle : Inport  Port=7
  muRoad : Inport  Port=8
  Ground{1..11} (11 alike) : Ground
  Terminator{,1..6,12} (8 alike) : Terminator
  Slp : Outport  VectorParamsAs1DForOutWhenUnconnected=off
  Alpha : Outport  Port=2  VectorParamsAs1DForOutWhenUnconnected=off
  TurnSlp : Outport  Port=3  VectorParamsAs1DForOutWhenUnconnected=off
  rBelt_eff : Outport  Port=4  VectorParamsAs1DForOutWhenUnconnected=off
  vBelt : Outport  Port=5  VectorParamsAs1DForOutWhenUnconnected=off
  LongFrc : Outport  Port=6  VectorParamsAs1DForOutWhenUnconnected=off
  SideFrc : Outport  Port=7  VectorParamsAs1DForOutWhenUnconnected=off
  LoadFrc : Outport  Port=8  VectorParamsAs1DForOutWhenUnconnected=off
  OverturnTrq : Outport  Port=9  VectorParamsAs1DForOutWhenUnconnected=off
  RollResist : Outport  Port=10  VectorParamsAs1DForOutWhenUnconnected=off
  AlignTrq : Outport  Port=11  VectorParamsAs1DForOutWhenUnconnected=off
  wires:
  Ground11/1 -> vBelt/1
  Ground10/1 -> rBelt_eff/1
  Ground9/1 -> TurnSlp/1
  Rim_turnv/1 -> Terminator6/1
  Sync_In/1 -> Terminator12/1
  Ground2/1 -> Alpha/1
  Ground3/1 -> LongFrc/1
  Ground4/1 -> SideFrc/1
  Ground5/1 -> OverturnTrq/1
  vxtrans/1 -> Terminator1/1
  vytrans/1 -> Terminator2/1
  Rim_rotv/1 -> Terminator3/1
  InclinAngle/1 -> Terminator4/1
  muRoad/1 -> Terminator5/1
  Load/1 -> Terminator/1
  Ground1/1 -> Slp/1
  Ground6/1 -> LoadFrc/1
  Ground7/1 -> RollResist/1
  Ground8/1 -> AlignTrq/1

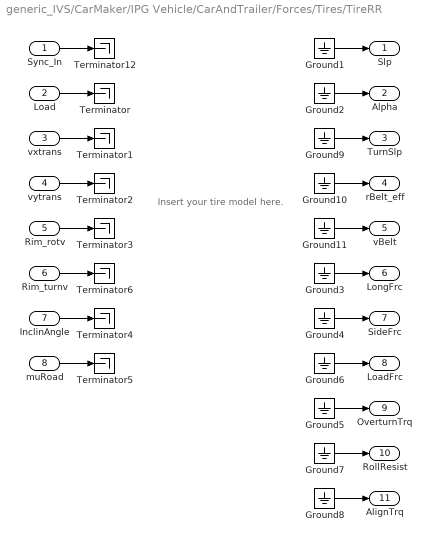
== system generic_IVS/CarMaker/IPG Vehicle/CarAndTrailer/Forces/Tires/TireRR ==
  note: Insert your tire model here.
  Sync_In : Inport
  Load : Inport  Port=2
  vxtrans : Inport  Port=3
  vytrans : Inport  Port=4
  Rim_rotv : Inport  Port=5
  Rim_turnv : Inport  Port=6
  InclinAngle : Inport  Port=7
  muRoad : Inport  Port=8
  Ground{1..11} (11 alike) : Ground
  Terminator{,1..6,12} (8 alike) : Terminator
  Slp : Outport  VectorParamsAs1DForOutWhenUnconnected=off
  Alpha : Outport  Port=2  VectorParamsAs1DForOutWhenUnconnected=off
  TurnSlp : Outport  Port=3  VectorParamsAs1DForOutWhenUnconnected=off
  rBelt_eff : Outport  Port=4  VectorParamsAs1DForOutWhenUnconnected=off
  vBelt : Outport  Port=5  VectorParamsAs1DForOutWhenUnconnected=off
  LongFrc : Outport  Port=6  VectorParamsAs1DForOutWhenUnconnected=off
  SideFrc : Outport  Port=7  VectorParamsAs1DForOutWhenUnconnected=off
  LoadFrc : Outport  Port=8  VectorParamsAs1DForOutWhenUnconnected=off
  OverturnTrq : Outport  Port=9  VectorParamsAs1DForOutWhenUnconnected=off
  RollResist : Outport  Port=10  VectorParamsAs1DForOutWhenUnconnected=off
  AlignTrq : Outport  Port=11  VectorParamsAs1DForOutWhenUnconnected=off
  wires:
  Ground11/1 -> vBelt/1
  Ground10/1 -> rBelt_eff/1
  Ground9/1 -> TurnSlp/1
  Rim_turnv/1 -> Terminator6/1
  Sync_In/1 -> Terminator12/1
  Ground2/1 -> Alpha/1
  Ground3/1 -> LongFrc/1
  Ground4/1 -> SideFrc/1
  Ground5/1 -> OverturnTrq/1
  vxtrans/1 -> Terminator1/1
  vytrans/1 -> Terminator2/1
  Rim_rotv/1 -> Terminator3/1
  InclinAngle/1 -> Terminator4/1
  muRoad/1 -> Terminator5/1
  Load/1 -> Terminator/1
  Ground1/1 -> Slp/1
  Ground6/1 -> LoadFrc/1
  Ground7/1 -> RollResist/1
  Ground8/1 -> AlignTrq/1

== matlab function generic_IVS/CarMaker/Subsystem/Final Project/Scenario 1/MATLAB Function11 ==
  settings: updateMethod=DISCRETE  sampleTime=0.05
  data: obstacle_info input; start_point input; goal_point input; x_path output; y_path output; is_reverse_path output
function [x_path, y_path, is_reverse_path] = rrt_path_planner(obstacle_info, start_point, goal_point)
%#codegen
    persistent success_cached x_path_cached y_path_cached is_reverse_path_cached
    MAX_PATH_LEN = 500;
    goal_point1 = [35,-8];
    goal_point2 = goal_point;
    %--- 캐시 초기화 및 반환 로직 ---
    if isempty(success_cached)
        % 처음 호출될 때
        success_cached  = false;
        x_path_cached   = zeros(MAX_PATH_LEN,1);
        y_path_cached   = zeros(MAX_PATH_LEN,1);
        is_reverse_path_cached = zeros(MAX_PATH_LEN, 1, 'logical');
        
    elseif success_cached
        % 이미 성공적으로 계산된 경로가 있으면 바로 반환
        x_path = x_path_cached;
        y_path = y_path_cached;
        is_reverse_path = is_reverse_path_cached;
        
        return;
    end

    %%RRT*
    MAX_NODES    = 2000;
    goal_radius  = 3.0;
    goal_sample_rate = 0.15;
    eta          = 2.0;

    start = [start_point(1), start_point(2)];
    finish_point  = goal_point1;
    vehicle_h_w = [1.47, 3.1];
    %vehicle_h_w = [2.1, 4.6];
    map_boundary = [5.5, -4, 47.5, -3.9, 47.5, -44.9, 5.5, -44.9];
    x_vals = map_boundary(1:2:end);
    y_vals = map_boundary(2:2:end);
    x_min = min(x_vals); x_max = max(x_vals);
    y_min = min(y_vals); y_max = max(y_vals);

    % 장애물 정보 파싱 (5개씩)
    if mod(length(obstacle_info),5) ~= 0
        obstacles = zeros(0,5);
    else
        num_obj = int32(floor(length(obstacle_info)/5));
        data = reshape(obstacle_info,[5, num_obj])';
        obstacles = [data(:,1), data(:,2), data(:,5), data(:,4), data(:,3)];
    end

    empty_node = struct('pos',zeros(1,2),'cost',0,'parent',int32(0));
    nodes = repmat(empty_node, MAX_NODES, 1);
    nodes(1).pos = start;
    node_count = int32(1);
    goal_node  = int32(0);

    % 샘플링 반복
    for iter = 1:2000
        if rand < goal_sample_rate
            sample = finish_point;
        else
            sample = [x_min + rand*(x_max-x_min), y_min + rand*(y_max-y_min)];
        end
        % 최근접 노드 찾기
        nearest_idx = int32(1);
        min_dist = norm(nodes(1).pos - sample);
        for i = 2:node_count
            d = norm(nodes(i).pos - sample);
            if d < min_dist
                min_dist = d;
                nearest_idx = int32(i);
            end
        end
        % 새 노드 생성
        dir_vec = sample - nodes(nearest_idx).pos;
        dist = norm(dir_vec);
        if dist > eta
            dir_vec = dir_vec / dist * eta;
        end
        new_pos = nodes(nearest_idx).pos + dir_vec;
        % 충돌 체크
        if check_collision(nodes(nearest_idx).pos, new_pos, vehicle_h_w, obstacles)
            continue;
        end
        % 노드 추가
        node_count = node_count + 1;
        if node_count > MAX_NODES, break; end
        nodes(node_count).pos    = new_pos;
        nodes(node_count).cost   = nodes(nearest_idx).cost + dist;
        nodes(node_count).parent = nearest_idx;
        % 목표 반경 체크
        if norm(new_pos - finish_point) < goal_radius
            goal_node = node_count;
            break;
        end
    end

    if goal_node > 0
        idx = goal_node; i = 0;
        temp_path = zeros(MAX_PATH_LEN,2);
        while idx>0 && i<MAX_PATH_LEN
            i = i + 1;
            temp_path(i,:) = nodes(idx).pos;
            idx = nodes(idx).parent;
        end
        flipped = flipud(temp_path(1:i,:));
     %% 후진 주차 segment 생성
        % % goal_point2 = goal_point;        % 엉덩이 기준
        % goal_point2 = [17,-9];
        % goal_yaw    = -pi/2;
        % vehicle_L   = vehicle_h_w(2);  % 차량 길이
        % goal_center = goal_point2 + (vehicle_L/2) * [cos(goal_yaw), sin(goal_yaw)];
        % 
        % direction_vec = goal_center - flipped(end,:);  % 실제 후진 벡터
        % expected_vec = [cos(goal_yaw), sin(goal_yaw)];
        % if dot(direction_vec, expected_vec) > 0  % 방향이 같다면 반전 필요
        %     goal_yaw = wrapToPi(goal_yaw + pi);
        % end
        % % 후진 경로 생성 (goal_point1 → goal_point2 방향)
        % step_size = 0.5;
        % reverse_dist = norm(goal_center - flipped(end,:));
        % num_steps = ceil(reverse_dist / step_size);
        % 
        % reverse_path = zeros(num_steps, 2);
        % for k = 1:num_steps
        %     reverse_path(k,:) = goal_center + (step_size * (num_steps - k)) * [-cos(goal_yaw), -sin(goal_yaw)];
        % end
        
        reverse_path = generate_rrt_segment(goal_point1, goal_point2, vehicle_h_w, obstacles, map_boundary);
        

        % 전체 raw path 구성
        raw_path = [flipped; reverse_path];
        is_reverse_path = zeros(MAX_PATH_LEN, 1, 'logical');
        reverse_start_idx = size(flipped, 1) + 1;
        reverse_len = size(reverse_path, 1);
        is_reverse_path(reverse_start_idx : reverse_start_idx + reverse_len - 1) = true;
        % pre_steps  = 10; post_steps = 8; step_dist = 0.5;
        % last_pos = flipped(end,:);
        % if last_pos(1) < finish_point(1)
        %     hybrid_x = finish_point(1) - 0.9;
        % else
        %     hybrid_x = finish_point(1) + 0.9;
        % end
        % if finish_point(2) > -36.5
        %     pre_path  = [ repmat(hybrid_x,pre_steps,1), finish_point(2)-step_dist*(pre_steps:-1:1)'];
        %     post_path = [ repmat(hybrid_x,post_steps,1), finish_point(2)+step_dist*(1:post_steps)' ];
        % else
        %     pre_path  = [ repmat(hybrid_x,pre_steps,1), finish_point(2)+step_dist*(pre_steps:-1:1)'];
        %     post_path = [ repmat(hybrid_x,post_steps,1), finish_point(2)-step_dist*(1:post_steps)' ];
        % end
        % hybrid_path = [pre_path; finish_point; post_path];
        % 
        % raw_path   = [flipped; hybrid_path];

        path_interp = smooth_path(raw_path, 0.5);
        path_interp = smooth_moving_average(path_interp, 20);

        % 최종 경로
        path_len = size(path_interp,1);
        path_out = zeros(MAX_PATH_LEN,2);
        path_out(1:path_len,:) = path_interp;

        % x,y 분리 및 캐싱
        x_path = path_out(:,1);
        y_path = path_out(:,2);
        x_path_cached  = x_path;
        y_path_cached  = y_path;
        is_reverse_path_cached = is_reverse_path; 
        success_cached = true;
    else
        % 실패 시 빈 벡터
        x_path = zeros(MAX_PATH_LEN,1);
        y_path = zeros(MAX_PATH_LEN,1);
        is_reverse_path = false(MAX_PATH_LEN,1);
    end
end

%% ===== 보조 함수
function collision = check_collision(p1, p2, vehicle_size, obs_list)
    collision = false;
    steps = 10;
    exception_obs = [26.5, -4, 0.1, 42.0, 0];
    for t = linspace(0,1,steps)
        pt = (1-t)*p1 + t*p2;
        yaw = atan2(p2(2)-p1(2), p2(1)-p1(1));
        veh = get_bbox(pt, yaw, vehicle_size);
        for i = 1:size(obs_list,1)
            if check_single_collision(veh, obs_list(i,:))
                collision = true; return;
            end
        end
        if check_single_collision(veh, exception_obs)
            collision = true; return;
        end
    end
end

function smoothed = smooth_moving_average(path, windowSize)
    N = size(path,1);
    half = floor(windowSize/2);
    smoothed = zeros(N,2);

    for i = 1:N
        if i == 1 || i == N
            smoothed(i,:) = path(i,:);  % 시작점과 끝점은 고정
        else
            i0 = max(1, i-half);
            i1 = min(N, i+half);
            smoothed(i,:) = mean(path(i0:i1,:), 1);
        end
    end
end

function is_collide = check_single_collision(veh_box, obs)
    yaw_obs = obs(5);
    rear_center = obs(1:2);
    length_obs = obs(4);
    width_obs = obs(3);
    fwd_vec = [cos(yaw_obs), sin(yaw_obs)];
    center = rear_center + (length_obs/2) * fwd_vec;
    obs_box = get_bbox(center, yaw_obs, [width_obs, length_obs]);
    is_collide = box_overlap(veh_box, obs_box);
end

function box = get_bbox(center, yaw, size)
    w = size(1); h = size(2);
    dx = [ w/2, -w/2, -w/2,  w/2];
    dy = [ h/2,  h/2, -h/2, -h/2];
    R = [cos(yaw), -sin(yaw); sin(yaw), cos(yaw)];
    temp = R * [dx; dy];
    box = temp + center';
end

function overlap = box_overlap(b1, b2)
    overlap = true;
    axes = get_axes(b1, b2);
    for i = 1:size(axes,2)
        proj1 = axes(:,i)' * b1;
        proj2 = axes(:,i)' * b2;
        if max(proj1) < min(proj2) || max(proj2) < min(proj1)
            overlap = false;
            return;
        end
    end
end

function axes = get_axes(b1, b2)
    edges = [b1(:,2)-b1(:,1), b1(:,3)-b1(:,2)];
    normals = [-edges(2,:); edges(1,:)];
    axes = normals ./ vecnorm(normals);
end

function path_smooth = smooth_path(path_raw, step_size)
    if size(path_raw, 1) < 2
        path_smooth = path_raw;
        return;
    end
    dist = [0; cumsum(vecnorm(diff(path_raw), 2, 2))];
    query = 0:step_size:dist(end);
    if query(end) < dist(end)
        query(end+1) = dist(end);
    end
    x_interp = spline(dist, path_raw(:,1), query);
    y_interp = spline(dist, path_raw(:,2), query);
    path_smooth = [x_interp', y_interp'];
end


%%
function path = generate_rrt_segment(start_point, end_point, vehicle_h_w, obstacles, map_boundary)
    MAX_NODES    = 1000;
    goal_radius  = 10.0;
    goal_sample_rate = 0.3;
    eta          = 3.0;

    x_min = min(start_point(1), end_point(1)) - 2;
    x_max = max(start_point(1), end_point(1)) + 2;
    y_min = min(start_point(2), end_point(2)) - 2;
    y_max = max(start_point(2), end_point(2)) + 2;

    % 노드 초기화
    empty_node.pos    = zeros(1, 2);
    empty_node.cost   = 0;
    empty_node.parent = int32(0);
    nodes = repmat(empty_node, MAX_NODES, 1);
    nodes(1).pos = start_point;
    node_count = int32(1);
    goal_node = int32(0);

    for iter = 1:1500
        if rand < goal_sample_rate
            sample = end_point;
        else
            sample = [x_min + rand*(x_max-x_min), y_min + rand*(y_max-y_min)];
        end

        % 최근접 노드
        nearest_idx = int32(1);
        min_dist = norm(nodes(1).pos - sample);
        for i = 2:node_count
            d = norm(nodes(i).pos - sample);
            if d < min_dist
                min_dist = d;
                nearest_idx = int32(i);
            end
        end

        dir_vec = sample - nodes(nearest_idx).pos;
        dist = norm(dir_vec);
        if dist > eta
            dir_vec = dir_vec / dist * eta;
        end
        tmp = nodes(nearest_idx).pos + dir_vec;
        new_pos = zeros(1,2);
        new_pos(1) = tmp(1);
        new_pos(2) = tmp(2);

        % 충돌 체크
        if check_collision(nodes(nearest_idx).pos, new_pos, vehicle_h_w, obstacles)
            continue;
        end

        % 노드 추가
        node_count = node_count + 1;
        if node_count > MAX_NODES, break; end
        nodes(node_count).pos    = new_pos;
        nodes(node_count).cost   = nodes(nearest_idx).cost + dist;
        nodes(node_count).parent = nearest_idx;

        if norm(new_pos - end_point) < goal_radius
            goal_node = node_count;
            break;
        end
    end

    % 경로 추적
    MAX_PATH_LEN = 500;
    path = zeros(MAX_PATH_LEN, 2);
    n_path = 0;
    if goal_node > 0
        idx = goal_node;
        while idx > 0 && n_path < MAX_PATH_LEN
            n_path = n_path + 1;
            path(n_path, :) = nodes(idx).pos;
            idx = nodes(idx).parent;
        end
        path = flipud(path(1:n_path, :));  % 유효 경로만 반환
    else
        disp('[generate_rrt_segment] Failed');  % 디버그 로그
        path = zeros(0, 2);  % 실패 시 빈 경로
        return;
    end
end
